simulink model "upr_1_4"  (R2019a)
settings: Solver=VariableStepAuto  StartTime=0.0  StopTime=10.0  RelTol=1e-3
values from neighbouring files (symbols this model uses):
  Kp = 1    [1upr.m]    (also in upr_1.m)
  Td = 3    [1upr.m]    (also in PIDtun_CC.m = L*(0.37-0.37*tau)/(1-0.81*tau); PIDtun_ZN1.m = L/2; PIDtun_ZN2.m = 0.125*Tu; upr_1.m = 0.04)
  Ti = 0.5    [1upr.m]    (also in PIDtun_CC.m = L*(2.5-2*tau)/(1-0.39*tau); PIDtun_ZN1.m = 2*L; PIDtun_ZN2.m = 0.5*Tu; upr_1.m = 0.2)
settings Model: Creator=user1  LastModifiedBy=user1

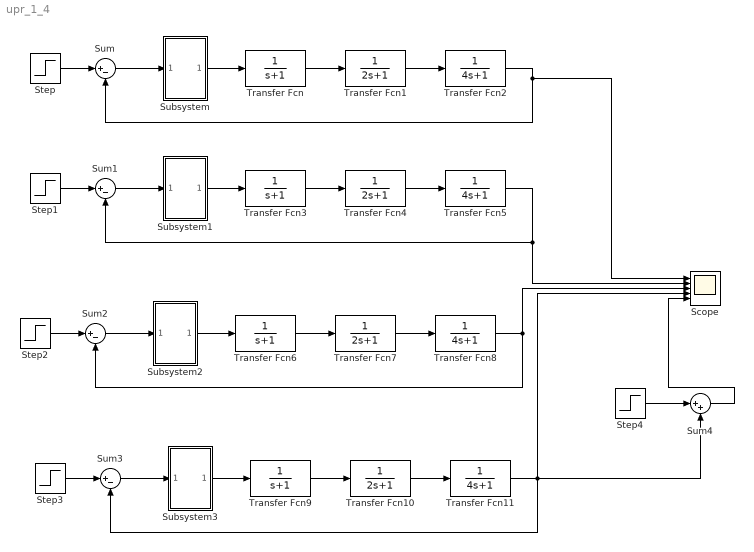
== system upr_1_4 ==
  Scope : Scope  NumInputPorts=5
  Step{,1..4} (5 alike) : Step  SampleTime=0
  Subsystem : Subsystem
  Subsystem1 : Subsystem
  Subsystem2 : Subsystem
  Subsystem3 : Subsystem
  Sum{,1..3} (4 alike) : Sum  Inputs=|+-
  Sum4 : Sum  Inputs=|++
  Transfer Fcn{,3,6,9} (4 alike) : TransferFcn  Denominator=[1 1]
  Transfer Fcn{1,4,7,10} (4 alike) : TransferFcn  Denominator=[2 1]
  Transfer Fcn{2,5,8,11} (4 alike) : TransferFcn  Denominator=[4 1]
  wires:
  Sum/1 -> Subsystem/1(In1)
  Transfer Fcn1/1 -> Transfer Fcn2/1
  Transfer Fcn2/1 -> Scope/1, Sum/2
  Step/1 -> Sum/1
  Transfer Fcn/1 -> Transfer Fcn1/1
  Sum1/1 -> Subsystem1/1(In1)
  Transfer Fcn4/1 -> Transfer Fcn5/1
  Transfer Fcn5/1 -> Scope/2, Sum1/2
  Step1/1 -> Sum1/1
  Transfer Fcn3/1 -> Transfer Fcn4/1
  Sum2/1 -> Subsystem2/1(In1)
  Transfer Fcn7/1 -> Transfer Fcn8/1
  Transfer Fcn8/1 -> Sum2/2, Scope/3
  Step2/1 -> Sum2/1
  Transfer Fcn6/1 -> Transfer Fcn7/1
  Sum3/1 -> Subsystem3/1(In1)
  Transfer Fcn10/1 -> Transfer Fcn11/1
  Transfer Fcn11/1 -> Sum4/2, Sum3/2, Scope/4
  Step3/1 -> Sum3/1
  Transfer Fcn9/1 -> Transfer Fcn10/1
  Step4/1 -> Sum4/1
  Sum4/1 -> Scope/5
  Subsystem/1(Out1) -> Transfer Fcn/1
  Subsystem1/1(Out1) -> Transfer Fcn3/1
  Subsystem2/1(Out1) -> Transfer Fcn6/1
  Subsystem3/1(Out1) -> Transfer Fcn9/1

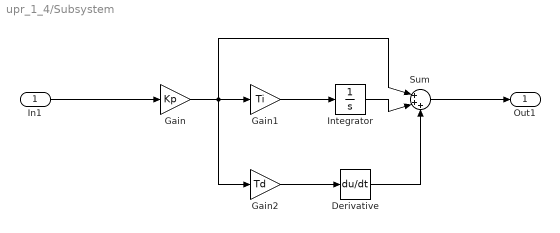
== system upr_1_4/Subsystem ==
  In1 : Inport
  Derivative : Derivative
  Gain : Gain  Gain=Kp
  Gain1 : Gain  Gain=Ti
  Gain2 : Gain  Gain=Td
  Integrator : Integrator
  Sum : Sum  Inputs=|+++
  Out1 : Outport
  wires:
  Gain1/1 -> Integrator/1
  Sum/1 -> Out1/1
  Gain/1 -> Sum/1, Gain2/1, Gain1/1
  In1/1 -> Gain/1
  Derivative/1 -> Sum/3
  Integrator/1 -> Sum/2
  Gain2/1 -> Derivative/1

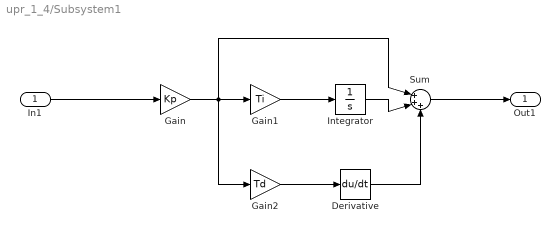
== system upr_1_4/Subsystem1 ==
  In1 : Inport
  Derivative : Derivative
  Gain : Gain  Gain=Kp
  Gain1 : Gain  Gain=Ti
  Gain2 : Gain  Gain=Td
  Integrator : Integrator
  Sum : Sum  Inputs=|+++
  Out1 : Outport
  wires:
  Gain1/1 -> Integrator/1
  Sum/1 -> Out1/1
  Gain/1 -> Sum/1, Gain2/1, Gain1/1
  In1/1 -> Gain/1
  Derivative/1 -> Sum/3
  Integrator/1 -> Sum/2
  Gain2/1 -> Derivative/1

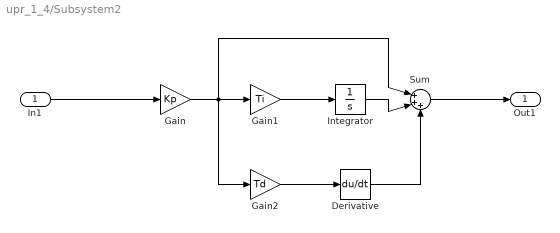
== system upr_1_4/Subsystem2 ==
  In1 : Inport
  Derivative : Derivative
  Gain : Gain  Gain=Kp
  Gain1 : Gain  Gain=Ti
  Gain2 : Gain  Gain=Td
  Integrator : Integrator
  Sum : Sum  Inputs=|+++
  Out1 : Outport
  wires:
  Gain1/1 -> Integrator/1
  Sum/1 -> Out1/1
  Gain/1 -> Sum/1, Gain2/1, Gain1/1
  In1/1 -> Gain/1
  Derivative/1 -> Sum/3
  Integrator/1 -> Sum/2
  Gain2/1 -> Derivative/1

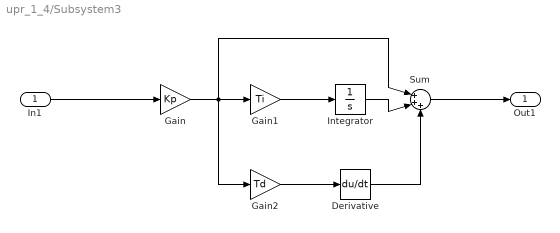
== system upr_1_4/Subsystem3 ==
  In1 : Inport
  Derivative : Derivative
  Gain : Gain  Gain=Kp
  Gain1 : Gain  Gain=Ti
  Gain2 : Gain  Gain=Td
  Integrator : Integrator
  Sum : Sum  Inputs=|+++
  Out1 : Outport
  wires:
  Gain1/1 -> Integrator/1
  Sum/1 -> Out1/1
  Gain/1 -> Sum/1, Gain2/1, Gain1/1
  In1/1 -> Gain/1
  Derivative/1 -> Sum/3
  Integrator/1 -> Sum/2
  Gain2/1 -> Derivative/1
